simulink model "MultiLoop_mode3"  (Simulink 10.0)
settings: Solver=ode45  StartTime=0.0  StopTime=72  FixedStep=Ts_base  MinStep=1e-6  RelTol=1e-6
values from neighbouring files (symbols this model uses):
  xInitial = xFinal    [prepNextSimIteration.m]
undefined symbols (not defined in the file or in its folder): idv_init, integrator_init, r1_0, r4_0, seed, Ts_base, Ts_save, xmv_0
undefined symbols (not defined in the file): Eadj_0, r5_0, r7_0, setpoint_change_duration, setpoint_init, SP17_0
libraries: simulink x12, TElib x10
settings Model: Creator=ricker  LastModifiedBy=christopher
settings DataIOCC: LoadInitialState=on  SaveFinalState=on  SaveFormat=Structure  SignalLoggingSaveFormat=ModelDataLogs  SaveOutput=off  SaveTime=off  SignalLoggingName=sigsOut
settings OptimizationCC: InitFltsAndDblsToZero=on
settings DebuggingCC: SaveWithParameterizedLinksMsg=none  SignalResolutionControl=TryResolveAllWithWarning  MultiTaskDSMMsg=warning  MultiTaskCondExecSysMsg=none  FcnCallInpInsideContextMsg=warning
settings HardwareCC: TargetUnknown=on
settings GRTTargetCC: TargetFcnLib=ansi_tfl_tmw.mat  GeneratePreprocessorConditionals=Disable all
settings ConfigComp: CovExternalEMLEnable=off  CovSFcnEnable=off

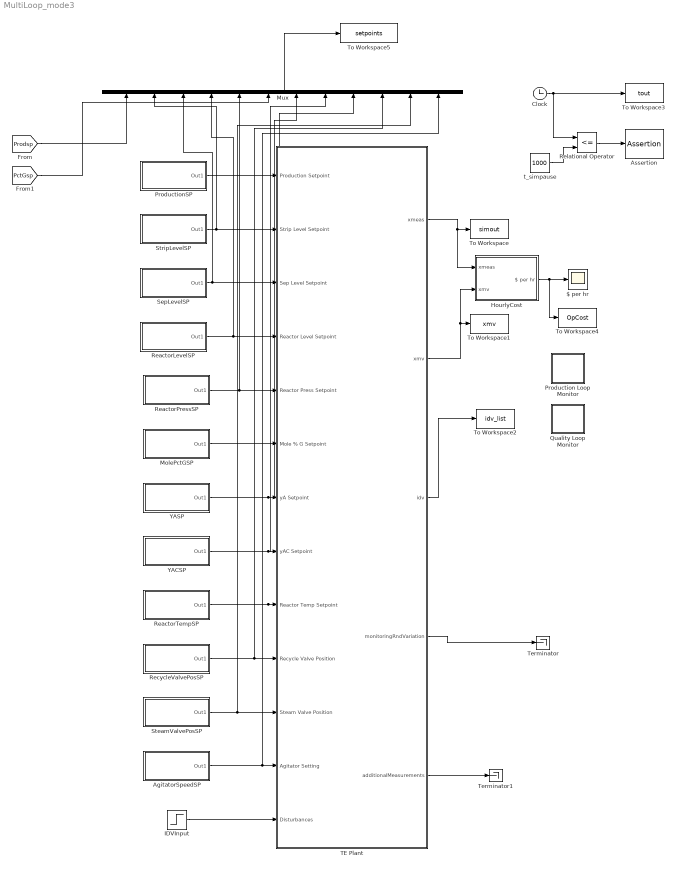
== system MultiLoop_mode3 ==
  $ per hr : Scope
  AgitatorSpeedSP : Subsystem  mask{SP_before=setpoint_init(1,12), SP_after=setpoint_init(2,12), tRampStart=setpoint_init(3,12), deltaT_ramp=setpoint_change_duration}
      mask prompts: SP_before "Value before ramp"; SP_after "Value after ramp"; tRampStart "Ramp start time"; deltaT_ramp "Ramp transition time"
  Assertion : Assertion  AssertionFailFcn=set_param(gcs ,'SimulationCommand','pause')  StopWhenAssertionFail=off
  Clock : Clock
  HourlyCost : Subsystem
  IDVInput : Step  Time=idv_init(3,:)  Before=idv_init(1,:)  After=idv_init(2,:)  SampleTime=0
  MolePctGSP : Subsystem  mask{SP_before=setpoint_init(1,6), SP_after=setpoint_init(2,6), tRampStart=setpoint_init(3,6), deltaT_ramp=setpoint_change_duration}
      mask prompts: SP_before "Value before ramp"; SP_after "Value after ramp"; tRampStart "Ramp start time"; deltaT_ramp "Ramp transition time"
  Mux : Mux  Inputs=12
  Production Loop Monitor : Subsystem
  ProductionSP : Subsystem  mask{SP_before=setpoint_init(1,1), SP_after=setpoint_init(2,1), tRampStart=setpoint_init(3,1), deltaT_ramp=setpoint_change_duration}
      mask prompts: SP_before "Value before ramp"; SP_after "Value after ramp"; tRampStart "Ramp start time"; deltaT_ramp "Ramp transition time"
  Quality Loop Monitor : Subsystem
  ReactorLevelSP : Subsystem  mask{SP_before=setpoint_init(1,4), SP_after=setpoint_init(2,4), tRampStart=setpoint_init(3,4), deltaT_ramp=setpoint_change_duration}
      mask prompts: SP_before "Value before ramp"; SP_after "Value after ramp"; tRampStart "Ramp start time"; deltaT_ramp "Ramp transition time"
  ReactorPressSP : Subsystem  mask{SP_before=setpoint_init(1,5), SP_after=setpoint_init(2,5), tRampStart=setpoint_init(3,5), deltaT_ramp=setpoint_change_duration}
      mask prompts: SP_before "Value before ramp"; SP_after "Value after ramp"; tRampStart "Ramp start time"; deltaT_ramp "Ramp transition time"
  ReactorTempSP : Subsystem  mask{SP_before=setpoint_init(1,9), SP_after=setpoint_init(2,9), tRampStart=setpoint_init(3,9), deltaT_ramp=setpoint_change_duration}
      mask prompts: SP_before "Value before ramp"; SP_after "Value after ramp"; tRampStart "Ramp start time"; deltaT_ramp "Ramp transition time"
  RecycleValvePosSP : Subsystem  mask{SP_before=setpoint_init(1,10), SP_after=setpoint_init(2,10), tRampStart=setpoint_init(3,10), deltaT_ramp=setpoint_change_duration}
      mask prompts: SP_before "Value before ramp"; SP_after "Value after ramp"; tRampStart "Ramp start time"; deltaT_ramp "Ramp transition time"
  Relational Operator : RelationalOperator  Operator=<=  OutDataTypeStr=boolean  RndMeth=Simplest
  SepLevelSP : Subsystem  mask{SP_before=setpoint_init(1,3), SP_after=setpoint_init(2,3), tRampStart=setpoint_init(3,3), deltaT_ramp=setpoint_change_duration}
      mask prompts: SP_before "Value before ramp"; SP_after "Value after ramp"; tRampStart "Ramp start time"; deltaT_ramp "Ramp transition time"
  SteamValvePosSP : Subsystem  mask{SP_before=setpoint_init(1,11), SP_after=setpoint_init(2,11), tRampStart=setpoint_init(3,11), deltaT_ramp=setpoint_change_duration}
      mask prompts: SP_before "Value before ramp"; SP_after "Value after ramp"; tRampStart "Ramp start time"; deltaT_ramp "Ramp transition time"
  StripLevelSP : Subsystem  mask{SP_before=setpoint_init(1,2), SP_after=setpoint_init(2,2), tRampStart=setpoint_init(3,2), deltaT_ramp=setpoint_change_duration}
      mask prompts: SP_before "Value before ramp"; SP_after "Value after ramp"; tRampStart "Ramp start time"; deltaT_ramp "Ramp transition time"
  TE Plant : Subsystem
  Terminator : Terminator
  Terminator1 : Terminator
  To Workspace : ToWorkspace  VariableName=simout  SampleTime=Ts_save
  To Workspace1 : ToWorkspace  VariableName=xmv  SampleTime=Ts_save
  To Workspace2 : ToWorkspace  VariableName=idv_list  SampleTime=Ts_save
  To Workspace3 : ToWorkspace  VariableName=tout  SampleTime=Ts_save
  To Workspace4 : ToWorkspace  VariableName=OpCost  SampleTime=Ts_save
  To Workspace5 : ToWorkspace  VariableName=setpoints  SampleTime=Ts_save
  YACSP : Subsystem  mask{SP_before=setpoint_init(1,8), SP_after=setpoint_init(2,8), tRampStart=setpoint_init(3,8), deltaT_ramp=setpoint_change_duration}
      mask prompts: SP_before "Value before ramp"; SP_after "Value after ramp"; tRampStart "Ramp start time"; deltaT_ramp "Ramp transition time"
  YASP : Subsystem  mask{SP_before=setpoint_init(1,7), SP_after=setpoint_init(2,7), tRampStart=setpoint_init(3,7), deltaT_ramp=setpoint_change_duration}
      mask prompts: SP_before "Value before ramp"; SP_after "Value after ramp"; tRampStart "Ramp start time"; deltaT_ramp "Ramp transition time"
  t_simpause : Constant  Value=1000
  wires:
  TE Plant/1(xmeas) -> HourlyCost/1(xmeas), To Workspace/1
  TE Plant/2(xmv) -> To Workspace1/1, HourlyCost/2(xmv)
  TE Plant/3(idv) -> To Workspace2/1
  Clock/1 -> Relational Operator/1, To Workspace3/1
  HourlyCost/1($ per hr) -> $ per hr/1, To Workspace4/1
  ProductionSP/1(Out1) -> TE Plant/1(Production Setpoint)
  AgitatorSpeedSP/1(Out1) -> Mux/12, TE Plant/12(Agitator Setting)
  SteamValvePosSP/1(Out1) -> Mux/11, TE Plant/11(Steam Valve Position)
  RecycleValvePosSP/1(Out1) -> Mux/10, TE Plant/10(Recycle Valve Position)
  ReactorTempSP/1(Out1) -> Mux/9, TE Plant/9(Reactor Temp Setpoint)
  YACSP/1(Out1) -> Mux/8, TE Plant/8(yAC Setpoint)
  YASP/1(Out1) -> Mux/7, TE Plant/7(yA Setpoint)
  MolePctGSP/1(Out1) -> TE Plant/6(Mole % G Setpoint)
  ReactorPressSP/1(Out1) -> TE Plant/5(Reactor Press Setpoint), Mux/5
  ReactorLevelSP/1(Out1) -> TE Plant/4(Reactor Level Setpoint), Mux/4
  SepLevelSP/1(Out1) -> TE Plant/3(Sep Level Setpoint), Mux/3
  StripLevelSP/1(Out1) -> TE Plant/2(Strip Level Setpoint), Mux/2
  IDVInput/1 -> TE Plant/13(Disturbances)
  Mux/1 -> To Workspace5/1
  TE Plant/4(monitoringRndVariation) -> Terminator/1
  TE Plant/5(additionalMeasurements) -> Terminator1/1
  [Prodsp] -> Mux/1
  [PctGsp] -> Mux/6
  Relational Operator/1 -> Assertion/1
  t_simpause/1 -> Relational Operator/2

== system MultiLoop_mode3/AgitatorSpeedSP ==
  Constant : Constant  Value=SP_before
  Constant1 : Constant  Value=deltaT_ramp
  Ramp : simulink/Sources/Ramp  slope=(SP_after-SP_before) /max(deltaT_ramp,0.1)  start=tRampStart  InitialOutput=0
  Saturation : Saturate  UpperLimit=max(SP_before, SP_after)  LowerLimit=min(SP_before, SP_after)
  Step : Step  Time=tRampStart  Before=SP_before  After=SP_after  SampleTime=0
  Sum : Sum  Inputs=|++
  Switch : Switch  Criteria=u2 > Threshold
  Out1 : Outport  VectorParamsAs1DForOutWhenUnconnected=off
  wires:
  Constant/1 -> Sum/1
  Ramp/1 -> Sum/2
  Sum/1 -> Saturation/1
  Constant1/1 -> Switch/2
  Switch/1 -> Out1/1
  Step/1 -> Switch/3
  Saturation/1 -> Switch/1

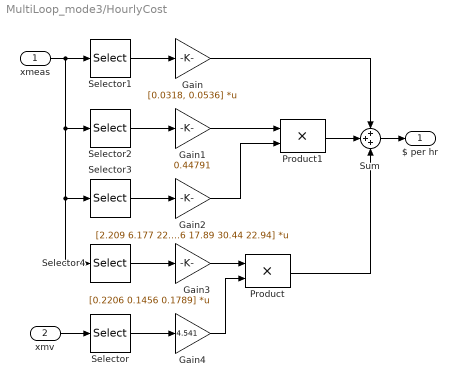
== system MultiLoop_mode3/HourlyCost ==
  xmeas : Inport  PortDimensions=41
  xmv : Inport  Port=2  PortDimensions=12
  Gain : Gain  Gain=[0.0318, 0.0536]  Multiplication=Matrix(K*u)  SaturateOnIntegerOverflow=on  OutDataTypeStr=Inherit: Same as input  ParamDataTypeStr=Inherit: Same as input
  Gain1 : Gain  Gain=0.44791  SaturateOnIntegerOverflow=on  OutDataTypeStr=Inherit: Same as input  ParamDataTypeStr=Inherit: Same as input
  Gain2 : Gain  Gain=[2.209 6.177 22.06 14.56 17.89 30.44 22.94]  Multiplication=Matrix(K*u)  SaturateOnIntegerOverflow=on  OutDataTypeStr=Inherit: Same as input  ParamDataTypeStr=Inherit: Same as input
  Gain3 : Gain  Gain=[0.2206 0.1456 0.1789]  Multiplication=Matrix(K*u)  SaturateOnIntegerOverflow=on  OutDataTypeStr=Inherit: Same as input  ParamDataTypeStr=Inherit: Same as input
  Gain4 : Gain  Gain=4.541  SaturateOnIntegerOverflow=on  OutDataTypeStr=Inherit: Same as input  ParamDataTypeStr=Inherit: Same as input
  Product : Product  SaturateOnIntegerOverflow=on  OutDataTypeStr=Inherit: Same as first input
  Product1 : Product  SaturateOnIntegerOverflow=on  OutDataTypeStr=Inherit: Same as first input
  Selector : Selector  InputPortWidth=12  IndexOptions=Index vector (dialog)  Indices=8  OutputSizes=1
  Selector1 : Selector  InputPortWidth=41  IndexOptions=Index vector (dialog)  Indices=[19 20]  OutputSizes=1
  Selector2 : Selector  InputPortWidth=41  IndexOptions=Index vector (dialog)  Indices=[10]  OutputSizes=1
  Selector3 : Selector  InputPortWidth=41  IndexOptions=Index vector (dialog)  Indices=[29, 31:36]  OutputSizes=1
  Selector4 : Selector  InputPortWidth=41  IndexOptions=Index vector (dialog)  Indices=[37:39]  OutputSizes=1
  Sum : Sum  Inputs=+++  SaturateOnIntegerOverflow=on
  $ per hr : Outport  VectorParamsAs1DForOutWhenUnconnected=off
  wires:
  xmv/1 -> Selector/1
  xmeas/1 -> Selector1/1, Selector2/1, Selector3/1, Selector4/1
  Selector1/1 -> Gain/1
  Selector2/1 -> Gain1/1
  Selector3/1 -> Gain2/1
  Selector4/1 -> Gain3/1
  Selector/1 -> Gain4/1
  Gain3/1 -> Product/1
  Gain4/1 -> Product/2
  Sum/1 -> $ per hr/1
  Product/1 -> Sum/3
  Gain/1 -> Sum/1
  Product1/1 -> Sum/2
  Gain1/1 -> Product1/1
  Gain2/1 -> Product1/2

== system MultiLoop_mode3/MolePctGSP ==
  Constant : Constant  Value=SP_before
  Constant1 : Constant  Value=deltaT_ramp
  Ramp : simulink/Sources/Ramp  slope=(SP_after-SP_before) /max(deltaT_ramp,0.1)  start=tRampStart  InitialOutput=0
  Saturation1 : Saturate  UpperLimit=max(SP_before, SP_after)  LowerLimit=min(SP_before, SP_after)
  Step : Step  Time=tRampStart  Before=SP_before  After=SP_after  SampleTime=0
  Sum : Sum  Inputs=|++
  Switch : Switch  Criteria=u2 > Threshold
  Out1 : Outport  VectorParamsAs1DForOutWhenUnconnected=off
  wires:
  Constant/1 -> Sum/1
  Ramp/1 -> Sum/2
  Sum/1 -> Saturation1/1
  Constant1/1 -> Switch/2
  Switch/1 -> Out1/1
  Step/1 -> Switch/3
  Saturation1/1 -> Switch/1

== system MultiLoop_mode3/Production Loop Monitor ==
  Mux2 : Mux  Inputs=2
  Production : Scope
  wires:
  Mux2/1 -> Production/1
  [xmeas17] -> Mux2/2
  [Prodsp] -> Mux2/1

== system MultiLoop_mode3/ProductionSP ==
  Constant : Constant  Value=SP_before
  Constant1 : Constant  Value=deltaT_ramp
  Ramp : simulink/Sources/Ramp  slope=(SP_after-SP_before) /max(deltaT_ramp,0.1)  start=tRampStart  InitialOutput=0
  Saturation : Saturate  UpperLimit=max(SP_before, SP_after)  LowerLimit=min(SP_before, SP_after)
  Step : Step  Time=tRampStart  Before=SP_before  After=SP_after  SampleTime=0
  Sum : Sum  Inputs=|++
  Switch : Switch  Criteria=u2 > Threshold
  Out1 : Outport  VectorParamsAs1DForOutWhenUnconnected=off
  wires:
  Constant/1 -> Sum/1
  Ramp/1 -> Sum/2
  Sum/1 -> Saturation/1
  Constant1/1 -> Switch/2
  Switch/1 -> Out1/1
  Step/1 -> Switch/3
  Saturation/1 -> Switch/1

== system MultiLoop_mode3/Quality Loop Monitor ==
  Mux2 : Mux  Inputs=2
  Quality : Scope
  wires:
  [PctGsp] -> Mux2/1
  [xmeas40] -> Mux2/2
  Mux2/1 -> Quality/1

== system MultiLoop_mode3/ReactorLevelSP ==
  Constant : Constant  Value=SP_before
  Constant1 : Constant  Value=deltaT_ramp
  Ramp : simulink/Sources/Ramp  slope=(SP_after-SP_before) /max(deltaT_ramp,0.1)  start=tRampStart  InitialOutput=0
  Saturation : Saturate  UpperLimit=max(SP_before, SP_after)  LowerLimit=min(SP_before, SP_after)
  Step : Step  Time=tRampStart  Before=SP_before  After=SP_after  SampleTime=0
  Sum : Sum  Inputs=|++
  Switch : Switch  Criteria=u2 > Threshold
  Out1 : Outport  VectorParamsAs1DForOutWhenUnconnected=off
  wires:
  Constant/1 -> Sum/1
  Ramp/1 -> Sum/2
  Sum/1 -> Saturation/1
  Constant1/1 -> Switch/2
  Switch/1 -> Out1/1
  Step/1 -> Switch/3
  Saturation/1 -> Switch/1

== system MultiLoop_mode3/ReactorPressSP ==
  Constant : Constant  Value=SP_before
  Constant1 : Constant  Value=deltaT_ramp
  Ramp : simulink/Sources/Ramp  slope=(SP_after-SP_before) /max(deltaT_ramp,0.1)  start=tRampStart  InitialOutput=0
  Saturation1 : Saturate  UpperLimit=max(SP_before, SP_after)  LowerLimit=min(SP_before, SP_after)
  Step : Step  Time=tRampStart  Before=SP_before  After=SP_after  SampleTime=0
  Sum : Sum  Inputs=|++
  Switch : Switch  Criteria=u2 > Threshold
  Out1 : Outport  VectorParamsAs1DForOutWhenUnconnected=off
  wires:
  Constant/1 -> Sum/1
  Ramp/1 -> Sum/2
  Sum/1 -> Saturation1/1
  Constant1/1 -> Switch/2
  Switch/1 -> Out1/1
  Step/1 -> Switch/3
  Saturation1/1 -> Switch/1

== system MultiLoop_mode3/ReactorTempSP ==
  Constant : Constant  Value=SP_before
  Constant1 : Constant  Value=deltaT_ramp
  Ramp : simulink/Sources/Ramp  slope=(SP_after-SP_before) /max(deltaT_ramp,0.1)  start=tRampStart  InitialOutput=0
  Saturation1 : Saturate  UpperLimit=max(SP_before, SP_after)  LowerLimit=min(SP_before, SP_after)
  Step : Step  Time=tRampStart  Before=SP_before  After=SP_after  SampleTime=0
  Sum : Sum  Inputs=|++
  Switch : Switch  Criteria=u2 > Threshold
  Out1 : Outport  VectorParamsAs1DForOutWhenUnconnected=off
  wires:
  Constant/1 -> Sum/1
  Ramp/1 -> Sum/2
  Sum/1 -> Saturation1/1
  Constant1/1 -> Switch/2
  Switch/1 -> Out1/1
  Step/1 -> Switch/3
  Saturation1/1 -> Switch/1

== system MultiLoop_mode3/RecycleValvePosSP ==
  Constant : Constant  Value=SP_before
  Constant1 : Constant  Value=deltaT_ramp
  Ramp : simulink/Sources/Ramp  slope=(SP_after-SP_before) /max(deltaT_ramp,0.1)  start=tRampStart  InitialOutput=0
  Saturation1 : Saturate  UpperLimit=max(SP_before, SP_after)  LowerLimit=min(SP_before, SP_after)
  Step : Step  Time=tRampStart  Before=SP_before  After=SP_after  SampleTime=0
  Sum : Sum  Inputs=|++
  Switch : Switch  Criteria=u2 > Threshold
  Out1 : Outport  VectorParamsAs1DForOutWhenUnconnected=off
  wires:
  Constant/1 -> Sum/1
  Ramp/1 -> Sum/2
  Sum/1 -> Saturation1/1
  Constant1/1 -> Switch/2
  Switch/1 -> Out1/1
  Step/1 -> Switch/3
  Saturation1/1 -> Switch/1

== system MultiLoop_mode3/SepLevelSP ==
  Constant : Constant  Value=SP_before
  Constant1 : Constant  Value=deltaT_ramp
  Ramp : simulink/Sources/Ramp  slope=(SP_after-SP_before) /max(deltaT_ramp,0.1)  start=tRampStart  InitialOutput=0
  Saturation1 : Saturate  UpperLimit=max(SP_before, SP_after)  LowerLimit=min(SP_before, SP_after)
  Step : Step  Time=tRampStart  Before=SP_before  After=SP_after  SampleTime=0
  Sum : Sum  Inputs=|++
  Switch : Switch  Criteria=u2 > Threshold
  Out1 : Outport  VectorParamsAs1DForOutWhenUnconnected=off
  wires:
  Constant/1 -> Sum/1
  Ramp/1 -> Sum/2
  Sum/1 -> Saturation1/1
  Constant1/1 -> Switch/2
  Switch/1 -> Out1/1
  Step/1 -> Switch/3
  Saturation1/1 -> Switch/1

== system MultiLoop_mode3/SteamValvePosSP ==
  Constant : Constant  Value=SP_before
  Constant1 : Constant  Value=deltaT_ramp
  Ramp : simulink/Sources/Ramp  slope=(SP_after-SP_before) /max(deltaT_ramp,0.1)  start=tRampStart  InitialOutput=0
  Saturation1 : Saturate  UpperLimit=max(SP_before, SP_after)  LowerLimit=min(SP_before, SP_after)
  Step : Step  Time=tRampStart  Before=SP_before  After=SP_after  SampleTime=0
  Sum : Sum  Inputs=|++
  Switch : Switch  Criteria=u2 > Threshold
  Out1 : Outport  VectorParamsAs1DForOutWhenUnconnected=off
  wires:
  Constant/1 -> Sum/1
  Ramp/1 -> Sum/2
  Sum/1 -> Saturation1/1
  Constant1/1 -> Switch/2
  Switch/1 -> Out1/1
  Step/1 -> Switch/3
  Saturation1/1 -> Switch/1

== system MultiLoop_mode3/StripLevelSP ==
  Constant : Constant  Value=SP_before
  Constant1 : Constant  Value=deltaT_ramp
  Ramp : simulink/Sources/Ramp  slope=(SP_after-SP_before) /max(deltaT_ramp,0.1)  start=tRampStart  InitialOutput=0
  Saturation : Saturate  UpperLimit=max(SP_before, SP_after)  LowerLimit=min(SP_before, SP_after)
  Step : Step  Time=tRampStart  Before=SP_before  After=SP_after  SampleTime=0
  Sum : Sum  Inputs=|++
  Switch : Switch  Criteria=u2 > Threshold
  Out1 : Outport  VectorParamsAs1DForOutWhenUnconnected=off
  wires:
  Constant/1 -> Sum/1
  Ramp/1 -> Sum/2
  Sum/1 -> Saturation/1
  Constant1/1 -> Switch/2
  Switch/1 -> Out1/1
  Step/1 -> Switch/3
  Saturation/1 -> Switch/1

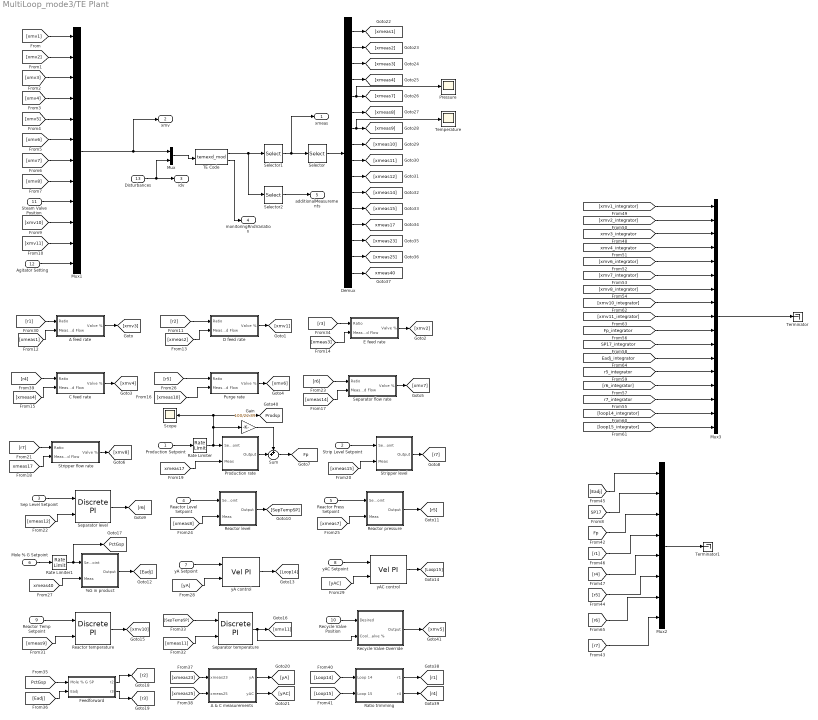
== system MultiLoop_mode3/TE Plant ==
  Production Setpoint : Inport
  Strip Level Setpoint : Inport  Port=2
  Sep Level Setpoint : Inport  Port=3
  Reactor Level Setpoint : Inport  Port=4
  Reactor Press Setpoint : Inport  Port=5
  Mole % G Setpoint : Inport  Port=6
  yA Setpoint : Inport  Port=7
  yAC Setpoint : Inport  Port=8
  Reactor Temp Setpoint : Inport  Port=9
  Recycle Valve Position : Inport  Port=10
  Steam Valve Position : Inport  Port=11
  Agitator Setting : Inport  Port=12
  Disturbances : Inport  Port=13
  %G in product : Subsystem  AncestorBlock=TElib/Discrete PI  mask{Kc=-0.4, Ti=100/60, Ts=Ts_base, x0=Eadj_0, Hi=inf, Lo=-inf}
  A & C measurements : Subsystem
  A feed rate : Subsystem
  C feed rate : Subsystem
  D feed rate : Subsystem
  Demux : Demux  Outputs=16
  E feed rate : Subsystem
  Feedforward : Subsystem
  Gain : Gain  Gain=100/22.89  SaturateOnIntegerOverflow=on  OutDataTypeStr=Inherit: Same as input  ParamDataTypeStr=Inherit: Same as input
  Mux : Mux  Inputs=2
  Mux1 : Mux  Inputs=12
  Mux2 : Mux  Inputs=8
  Mux3 : Mux  Inputs=17
  Pressure : Scope
  Production rate : Subsystem  AncestorBlock=TElib/Discrete PI  mask{Kc=3.2, Ti=120/60, Ts=Ts_base, x0=0, Hi=30, Lo=-30}
  Purge rate : Subsystem
  Rate Limiter : RateLimiter  RisingSlewLimit=0.3*22.95/24  FallingSlewLimit=-0.3*22.95/24
  Rate Limiter1 : RateLimiter  RisingSlewLimit=50/24  FallingSlewLimit=-50/24
  Ratio trimming : Subsystem
  Reactor level : Subsystem  AncestorBlock=TElib/Discrete PI  mask{Kc=0.8, Ti=60/60, Ts=Ts_base, x0=SP17_0, Hi=120, Lo=0}
  Reactor pressure : Subsystem  AncestorBlock=TElib/Discrete PI  mask{Kc=-1e-4, Ti=20/60, Ts=Ts_base, x0=r5_0, Hi=100, Lo=0}
  Reactor temperature : TElib/Discrete PI  Kc=-8  Ti=7.5/60  Ts=Ts_base  x0=xmv_0(10)  Hi=100  Lo=0
      link override Vel PI/Goto: GotoTag=xmv10_integrator
      link override Vel PI/Unit Delay: InitialCondition=integrator_init(8)
  Recycle Valve Override : Subsystem  AncestorBlock=TElib/Discrete PI
  Scope : Scope
  Selector : Selector  InputPortWidth=41  IndexOptions=Index vector (dialog)  Indices=[1:4, 7:12, 14, 15, 17, 23, 25, 40]  OutputSizes=1
  Selector1 : Selector  InputPortWidth=73  IndexOptions=Index vector (dialog)  Indices=[1:41]  OutputSizes=1
  Selector2 : Selector  InputPortWidth=73  IndexOptions=Index vector (dialog)  Indices=[42:73]  OutputSizes=1
  Separator flow rate : Subsystem
  Separator level : TElib/Discrete PI  Kc=-1e-3  Ti=200/60  Ts=Ts_base  x0=r6_0  Hi=100  Lo=0
      link override Vel PI/Goto: GotoTag=r6_integrator
      link override Vel PI/Unit Delay: InitialCondition=integrator_init(14)
  Separator temperature : TElib/Discrete PI  Kc=-4  Ti=15/60  Ts=Ts_base  x0=xmv_0(11)  Hi=100  Lo=0
      link override Vel PI/Goto: GotoTag=xmv11_integrator
      link override Vel PI/Unit Delay: InitialCondition=integrator_init(9)
  Stripper flow rate : Subsystem
  Stripper level : Subsystem  AncestorBlock=TElib/Discrete PI  mask{Kc=-2e-4, Ti=200/60, Ts=Ts_base, x0=r7_0, Hi=100, Lo=0}
  Sum : Sum  Inputs=++|  SaturateOnIntegerOverflow=on
  TE Code : S-Function  FunctionName=temexd_mod  Parameters=xInitial.signals(1).values,seed,243  SFunctionDeploymentMode=off  EnableBusSupport=off
  Temperature : Scope
  Terminator : Terminator
  Terminator1 : Terminator
  yA control : TElib/Discrete PI/Vel PI  Kc=2e-4  Ti=1  Ts=0.1
      link override Goto: GotoTag=loop14_integrator
      link override Unit Delay: InitialCondition=integrator_init(16)
  yAC control : TElib/Discrete PI/Vel PI  Kc=3e-4  Ti=2  Ts=0.1
      link override Goto: GotoTag=loop15_integrator
      link override Unit Delay: InitialCondition=integrator_init(17)
  xmeas : Outport  VectorParamsAs1DForOutWhenUnconnected=off
  xmv : Outport  Port=2  VectorParamsAs1DForOutWhenUnconnected=off
  idv : Outport  Port=3  VectorParamsAs1DForOutWhenUnconnected=off
  monitoringRndVariation : Outport  Port=4  VectorParamsAs1DForOutWhenUnconnected=off
  additionalMeasurements : Outport  Port=5  VectorParamsAs1DForOutWhenUnconnected=off
  tag scope: Fp=global, PctGsp=global, Prodsp=global, xmeas17=global, xmeas40=global
  wires:
  Mux/1 -> TE Code/1
  Disturbances/1 -> Mux/2, idv/1
  TE Code/1 -> Selector2/1, Selector1/1
  [xmv1] -> Mux1/1
  [xmv2] -> Mux1/2
  [xmv3] -> Mux1/3
  [xmv4] -> Mux1/4
  [xmv6] -> Mux1/6
  [xmv7] -> Mux1/7
  [xmv8] -> Mux1/8
  Steam Valve Position/1 -> Mux1/9
  [xmv10] -> Mux1/10
  [xmv11] -> Mux1/11
  Agitator Setting/1 -> Mux1/12
  A feed rate/1(Valve %) -> [xmv3]
  [xmeas1] -> A feed rate/2(Measured Flow)
  D feed rate/1(Valve %) -> [xmv1]
  [xmeas2] -> D feed rate/2(Measured Flow)
  E feed rate/1(Valve %) -> [xmv2]
  [xmeas3] -> E feed rate/2(Measured Flow)
  C feed rate/1(Valve %) -> [xmv4]
  [xmeas4] -> C feed rate/2(Measured Flow)
  Purge rate/1(Valve %) -> [xmv6]
  [xmeas10] -> Purge rate/2(Measured Flow)
  Separator flow rate/1(Valve %) -> [xmv7]
  [xmeas14] -> Separator flow rate/2(Measured Flow)
  Stripper flow rate/1(Valve %) -> [xmv8]
  [xmeas17] -> Stripper flow rate/2(Measured Flow)
  [xmeas17] -> Production rate/2(Meas)
  [xmeas15] -> Stripper level/2(Meas)
  Strip Level Setpoint/1 -> Stripper level/1(Setpoint)
  Stripper level/1(Output) -> [r7]
  [r7] -> Stripper flow rate/1(Ratio)
  [xmeas12] -> Separator level/2
  Sep Level Setpoint/1 -> Separator level/1
  Separator level/1 -> [r6]
  [r6] -> Separator flow rate/1(Ratio)
  [xmeas8] -> Reactor level/2(Meas)
  Reactor Level Setpoint/1 -> Reactor level/1(Setpoint)
  Reactor level/1(Output) -> [SepTempSP]
  [xmeas7] -> Reactor pressure/2(Meas)
  Reactor Press Setpoint/1 -> Reactor pressure/1(Setpoint)
  Reactor pressure/1(Output) -> [r5]
  [r5] -> Purge rate/1(Ratio)
  [xmeas40] -> %G in product/2(Meas)
  %G in product/1(Output) -> [Eadj]
  [yA] -> yA control/2
  yA Setpoint/1 -> yA control/1
  yA control/1 -> [Loop14]
  [yAC] -> yAC control/2
  yAC Setpoint/1 -> yAC control/1
  yAC control/1 -> [Loop15]
  [r1] -> A feed rate/1(Ratio)
  [xmeas9] -> Reactor temperature/2
  Reactor Temp Setpoint/1 -> Reactor temperature/1
  Reactor temperature/1 -> [xmv10]
  [xmeas11] -> Separator temperature/2
  [SepTempSP] -> Separator temperature/1
  Separator temperature/1 -> [xmv11], Recycle Valve Override/2(Coolant Valve %)
  [r2] -> D feed rate/1(Ratio)
  [r3] -> E feed rate/1(Ratio)
  [PctGsp] -> Feedforward/1(Mole % G SP)
  [Eadj] -> Feedforward/2(Eadj)
  Feedforward/1(r2) -> [r2]
  Feedforward/2(r3) -> [r3]
  [xmeas23] -> A & C measurements/1(xmeas23)
  [xmeas25] -> A & C measurements/2(xmeas25)
  A & C measurements/1(yA) -> [yA]
  A & C measurements/2(yAC) -> [yAC]
  Mux1/1 -> Mux/1, xmv/1
  Selector/1 -> Demux/1
  Demux/1 -> [xmeas1]
  Demux/2 -> [xmeas2]
  Demux/3 -> [xmeas3]
  Demux/4 -> [xmeas4]
  Demux/5 -> [xmeas7], Pressure/1
  Demux/6 -> [xmeas8]
  Demux/7 -> [xmeas9], Temperature/1
  Demux/8 -> [xmeas10]
  Demux/9 -> [xmeas11]
  Demux/10 -> [xmeas12]
  Demux/11 -> [xmeas14]
  Demux/12 -> [xmeas15]
  Demux/13 -> [xmeas17]
  Demux/14 -> [xmeas23]
  Demux/15 -> [xmeas25]
  Demux/16 -> [xmeas40]
  [r4] -> C feed rate/1(Ratio)
  [Loop14] -> Ratio trimming/1(Loop 14)
  [Loop15] -> Ratio trimming/2(Loop 15)
  Ratio trimming/1(r1) -> [r1]
  Ratio trimming/2(r4) -> [r4]
  Production Setpoint/1 -> Rate Limiter/1
  Rate Limiter/1 -> Production rate/1(Setpoint), Scope/1, [Prodsp], Gain/1
  Mole % G Setpoint/1 -> Rate Limiter1/1
  Rate Limiter1/1 -> %G in product/1(Setpoint), [PctGsp]
  Production rate/1(Output) -> Sum/2
  Sum/1 -> [Fp]
  Gain/1 -> Sum/1
  [xmv5] -> Mux1/5
  Recycle Valve Override/1(Output) -> [xmv5]
  Recycle Valve Position/1 -> Recycle Valve Override/1(Desired)
  Selector2/1 -> additionalMeasurements/1
  TE Code/2 -> monitoringRndVariation/1
  Selector1/1 -> xmeas/1, Selector/1
  [Eadj] -> Mux2/1
  [SP17] -> Mux2/2
  [Fp] -> Mux2/3
  [r1] -> Mux2/4
  [r4] -> Mux2/5
  [r5] -> Mux2/6
  [r7] -> Mux2/8
  [xmv1_integrator] -> Mux3/1
  [xmv2_integrator] -> Mux3/2
  [xmv3_integrator] -> Mux3/3
  [xmv4_integrator] -> Mux3/4
  [xmv6_integrator] -> Mux3/5
  [xmv7_integrator] -> Mux3/6
  [xmv8_integrator] -> Mux3/7
  [xmv10_integrator] -> Mux3/8
  [xmv11_integrator] -> Mux3/9
  [Fp_integrator] -> Mux3/10
  [SP17_integrator] -> Mux3/11
  [Eadj_integrator] -> Mux3/12
  [r5_integrator] -> Mux3/13
  [r6_integrator] -> Mux3/14
  [r7_integrator] -> Mux3/15
  [loop14_integrator] -> Mux3/16
  [loop15_integrator] -> Mux3/17
  [r6] -> Mux2/7
  Mux3/1 -> Terminator/1
  Mux2/1 -> Terminator1/1

== system MultiLoop_mode3/YACSP ==
  Constant : Constant  Value=SP_before
  Constant1 : Constant  Value=deltaT_ramp
  Ramp : simulink/Sources/Ramp  slope=(SP_after-SP_before) /max(deltaT_ramp,0.1)  start=tRampStart  InitialOutput=0
  Saturation1 : Saturate  UpperLimit=max(SP_before, SP_after)  LowerLimit=min(SP_before, SP_after)
  Step : Step  Time=tRampStart  Before=SP_before  After=SP_after  SampleTime=0
  Sum : Sum  Inputs=|++
  Switch : Switch  Criteria=u2 > Threshold
  Out1 : Outport  VectorParamsAs1DForOutWhenUnconnected=off
  wires:
  Constant/1 -> Sum/1
  Ramp/1 -> Sum/2
  Sum/1 -> Saturation1/1
  Constant1/1 -> Switch/2
  Switch/1 -> Out1/1
  Step/1 -> Switch/3
  Saturation1/1 -> Switch/1

== system MultiLoop_mode3/YASP ==
  Constant : Constant  Value=SP_before
  Constant1 : Constant  Value=deltaT_ramp
  Ramp : simulink/Sources/Ramp  slope=(SP_after-SP_before) /max(deltaT_ramp,0.1)  start=tRampStart  InitialOutput=0
  Saturation1 : Saturate  UpperLimit=max(SP_before, SP_after)  LowerLimit=min(SP_before, SP_after)
  Step : Step  Time=tRampStart  Before=SP_before  After=SP_after  SampleTime=0
  Sum : Sum  Inputs=|++
  Switch : Switch  Criteria=u2 > Threshold
  Out1 : Outport  VectorParamsAs1DForOutWhenUnconnected=off
  wires:
  Constant/1 -> Sum/1
  Ramp/1 -> Sum/2
  Sum/1 -> Saturation1/1
  Constant1/1 -> Switch/2
  Switch/1 -> Out1/1
  Step/1 -> Switch/3
  Saturation1/1 -> Switch/1

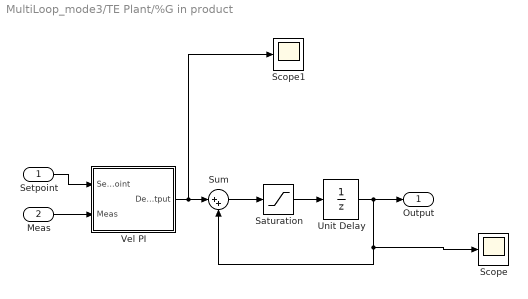
== system MultiLoop_mode3/TE Plant/%G in product ==
  Setpoint : Inport
  Meas : Inport  Port=2
  Saturation : Saturate  UpperLimit=Hi  LowerLimit=Lo
  Scope : Scope
  Scope1 : Scope
  Sum : Sum  Inputs=|++  SaturateOnIntegerOverflow=on
  Unit Delay : UnitDelay  InitialCondition=x0  SampleTime=Ts
  Vel PI : Subsystem  mask{Kc=Kc, Ti=Ti, Ts=Ts}
  Output : Outport
  wires:
  Setpoint/1 -> Vel PI/1(Setpoint)
  Meas/1 -> Vel PI/2(Meas)
  Unit Delay/1 -> Output/1, Scope/1, Sum/2
  Saturation/1 -> Unit Delay/1
  Vel PI/1(Delta Output) -> Scope1/1, Sum/1
  Sum/1 -> Saturation/1

== system MultiLoop_mode3/TE Plant/A & C measurements ==
  xmeas23 : Inport
  xmeas25 : Inport  Port=2
  Gain1 : Gain  Gain=100  SaturateOnIntegerOverflow=on  OutDataTypeStr=Inherit: Same as input  ParamDataTypeStr=Inherit: Same as input
  Product1 : Product  Inputs=*/  SaturateOnIntegerOverflow=on  OutDataTypeStr=Inherit: Same as first input
  Sum1 : Sum  Inputs=++|  SaturateOnIntegerOverflow=on
  yA : Outport  VectorParamsAs1DForOutWhenUnconnected=off
  yAC : Outport  Port=2  VectorParamsAs1DForOutWhenUnconnected=off
  wires:
  Sum1/1 -> yAC/1, Product1/2
  xmeas23/1 -> Sum1/1, Gain1/1
  xmeas25/1 -> Sum1/2
  Gain1/1 -> Product1/1
  Product1/1 -> yA/1

== system MultiLoop_mode3/TE Plant/A feed rate ==
  Ratio : Inport
  Measured Flow : Inport  Port=2
  Discrete PI : Subsystem  AncestorBlock=TElib/Discrete PI  mask{Kc=0.01, Ti=0.001/60, Ts=Ts_base, x0=xmv_0(3), Hi=100, Lo=0}
  Product : Product  SaturateOnIntegerOverflow=on  OutDataTypeStr=Inherit: Same as first input
  Scope : Scope
  Valve % : Outport  VectorParamsAs1DForOutWhenUnconnected=off
  wires:
  Discrete PI/1(Output) -> Valve %/1
  Ratio/1 -> Product/1
  [Fp] -> Product/2
  Measured Flow/1 -> Discrete PI/2(Meas)
  Product/1 -> Scope/1, Discrete PI/1(Setpoint)

== system MultiLoop_mode3/TE Plant/C feed rate ==
  Ratio : Inport
  Measured Flow : Inport  Port=2
  Discrete PI : Subsystem  AncestorBlock=TElib/Discrete PI  mask{Kc=0.003, Ti=0.001/60, Ts=Ts_base, x0=xmv_0(4), Hi=100, Lo=0}
  Product : Product  SaturateOnIntegerOverflow=on  OutDataTypeStr=Inherit: Same as first input
  Scope : Scope  NumInputPorts=2
  Valve % : Outport  VectorParamsAs1DForOutWhenUnconnected=off
  wires:
  Product/1 -> Scope/1, Discrete PI/1(Setpoint)
  Measured Flow/1 -> Scope/2, Discrete PI/2(Meas)
  [Fp] -> Product/2
  Ratio/1 -> Product/1
  Discrete PI/1(Output) -> Valve %/1

== system MultiLoop_mode3/TE Plant/D feed rate ==
  Ratio : Inport
  Measured Flow : Inport  Port=2
  Discrete PI : TElib/Discrete PI  Kc=1.6e-6  Ti=0.001/60  Ts=Ts_base  x0=xmv_0(1)  Hi=100  Lo=0
      link override Vel PI/Goto: GotoTag=xmv1_integrator
      link override Vel PI/Unit Delay: InitialCondition=integrator_init(1)
  Product : Product  SaturateOnIntegerOverflow=on  OutDataTypeStr=Inherit: Same as first input
  Valve % : Outport  VectorParamsAs1DForOutWhenUnconnected=off
  wires:
  Product/1 -> Discrete PI/1
  Measured Flow/1 -> Discrete PI/2
  [Fp] -> Product/2
  Ratio/1 -> Product/1
  Discrete PI/1 -> Valve %/1

== system MultiLoop_mode3/TE Plant/E feed rate ==
  Ratio : Inport
  Measured Flow : Inport  Port=2
  Discrete PI : TElib/Discrete PI  Kc=1.8e-6  Ti=0.001/60  Ts=Ts_base  x0=xmv_0(2)  Hi=100  Lo=0
      link override Vel PI/Goto: GotoTag=xmv2_integrator
      link override Vel PI/Unit Delay: InitialCondition=integrator_init(2)
  Product : Product  SaturateOnIntegerOverflow=on  OutDataTypeStr=Inherit: Same as first input
  Valve % : Outport  VectorParamsAs1DForOutWhenUnconnected=off
  wires:
  Product/1 -> Discrete PI/1
  Measured Flow/1 -> Discrete PI/2
  [Fp] -> Product/2
  Ratio/1 -> Product/1
  Discrete PI/1 -> Valve %/1

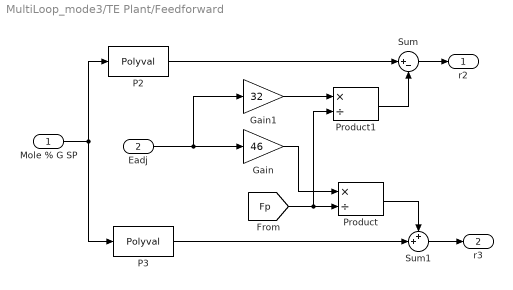
== system MultiLoop_mode3/TE Plant/Feedforward ==
  Mole % G SP : Inport
  Eadj : Inport  Port=2
  Gain : Gain  Gain=46  SaturateOnIntegerOverflow=on  OutDataTypeStr=Inherit: Same as input  ParamDataTypeStr=Inherit: Same as input
  Gain1 : Gain  Gain=32  SaturateOnIntegerOverflow=on  OutDataTypeStr=Inherit: Same as input  ParamDataTypeStr=Inherit: Same as input
  P2 : Polyval  Coefs="[1.5192e-003  5.9446e-001  2.7690e-001]"
  P3 : Polyval  Coefs="[-1.1377e-003 -8.0893e-001  9.1060e+001]"
  Product : Product  Inputs=*/  SaturateOnIntegerOverflow=on  OutDataTypeStr=Inherit: Same as first input
  Product1 : Product  Inputs=*/  SaturateOnIntegerOverflow=on  OutDataTypeStr=Inherit: Same as first input
  Sum : Sum  Inputs=|+-  SaturateOnIntegerOverflow=on
  Sum1 : Sum  Inputs=++|  SaturateOnIntegerOverflow=on
  r2 : Outport  VectorParamsAs1DForOutWhenUnconnected=off
  r3 : Outport  Port=2  VectorParamsAs1DForOutWhenUnconnected=off
  wires:
  Mole % G SP/1 -> P2/1, P3/1
  Sum/1 -> r2/1
  P2/1 -> Sum/1
  Sum1/1 -> r3/1
  P3/1 -> Sum1/2
  Product/1 -> Sum1/1
  [Fp] -> Product/2, Product1/2
  Gain/1 -> Product/1
  Eadj/1 -> Gain/1, Gain1/1
  Product1/1 -> Sum/2
  Gain1/1 -> Product1/1

== system MultiLoop_mode3/TE Plant/Production rate ==
  Setpoint : Inport
  Meas : Inport  Port=2
  Saturation : Saturate  UpperLimit=Hi  LowerLimit=Lo
  Sum : Sum  Inputs=|++  SaturateOnIntegerOverflow=on
  Unit Delay : UnitDelay  InitialCondition=x0  SampleTime=Ts
  Vel PI : Subsystem  mask{Kc=Kc, Ti=Ti, Ts=Ts}
  Output : Outport
  wires:
  Setpoint/1 -> Vel PI/1(Setpoint)
  Meas/1 -> Vel PI/2(Meas)
  Unit Delay/1 -> Output/1, Sum/2
  Saturation/1 -> Unit Delay/1
  Vel PI/1(Delta Output) -> Sum/1
  Sum/1 -> Saturation/1

== system MultiLoop_mode3/TE Plant/Purge rate ==
  Ratio : Inport
  Measured Flow : Inport  Port=2
  Discrete PI : TElib/Discrete PI  Kc=0.01  Ti=0.001/60  Ts=Ts_base  x0=xmv_0(6)  Hi=100  Lo=0
      link override Vel PI/Goto: GotoTag=xmv6_integrator
      link override Vel PI/Unit Delay: InitialCondition=integrator_init(5)
  Product : Product  SaturateOnIntegerOverflow=on  OutDataTypeStr=Inherit: Same as first input
  Valve % : Outport  VectorParamsAs1DForOutWhenUnconnected=off
  wires:
  Discrete PI/1 -> Valve %/1
  Ratio/1 -> Product/1
  [Fp] -> Product/2
  Measured Flow/1 -> Discrete PI/2
  Product/1 -> Discrete PI/1

== system MultiLoop_mode3/TE Plant/Ratio trimming ==
  Loop 14 : Inport
  Loop 15 : Inport  Port=2
  Sum1 : Sum  Inputs=-++  SaturateOnIntegerOverflow=on
  Sum2 : Sum  Inputs=++|  SaturateOnIntegerOverflow=on
  Unit Delay : UnitDelay  InitialCondition=r1_0  SampleTime=0.1  HasFrameUpgradeWarning=on
  Unit Delay1 : UnitDelay  InitialCondition=r4_0  SampleTime=0.1  HasFrameUpgradeWarning=on
  r1 : Outport  VectorParamsAs1DForOutWhenUnconnected=off
  r4 : Outport  Port=2  VectorParamsAs1DForOutWhenUnconnected=off
  wires:
  Loop 15/1 -> Sum1/2
  Unit Delay/1 -> Sum2/1
  Unit Delay1/1 -> Sum1/3
  Sum2/1 -> Unit Delay/1, r1/1
  Loop 14/1 -> Sum2/2, Sum1/1
  Sum1/1 -> Unit Delay1/1, r4/1

== system MultiLoop_mode3/TE Plant/Reactor level ==
  Setpoint : Inport
  Meas : Inport  Port=2
  Saturation : Saturate  UpperLimit=Hi  LowerLimit=Lo
  Sum : Sum  Inputs=|++  SaturateOnIntegerOverflow=on
  Unit Delay : UnitDelay  InitialCondition=x0  SampleTime=Ts
  Vel PI : Subsystem  mask{Kc=Kc, Ti=Ti, Ts=Ts}
  Output : Outport
  tag scope: SP17=global
  wires:
  Setpoint/1 -> Vel PI/1(Setpoint)
  Meas/1 -> Vel PI/2(Meas)
  Unit Delay/1 -> Output/1, Sum/2, [SP17]
  Saturation/1 -> Unit Delay/1
  Vel PI/1(Delta Output) -> Sum/1
  Sum/1 -> Saturation/1

== system MultiLoop_mode3/TE Plant/Reactor pressure ==
  Setpoint : Inport
  Meas : Inport  Port=2
  Saturation : Saturate  UpperLimit=Hi  LowerLimit=Lo
  Sum : Sum  Inputs=|++  SaturateOnIntegerOverflow=on
  Unit Delay : UnitDelay  InitialCondition=x0  SampleTime=Ts
  Vel PI : Subsystem  mask{Kc=Kc, Ti=Ti, Ts=Ts}
  Output : Outport
  wires:
  Setpoint/1 -> Vel PI/1(Setpoint)
  Meas/1 -> Vel PI/2(Meas)
  Unit Delay/1 -> Output/1, Sum/2
  Saturation/1 -> Unit Delay/1
  Vel PI/1(Delta Output) -> Sum/1
  Sum/1 -> Saturation/1

== system MultiLoop_mode3/TE Plant/Recycle Valve Override ==
  Desired : Inport
  Coolant Valve % : Inport  Port=2
  Gain : Gain  Gain=-2
  Max Allowed : Constant  Value=90
  Saturation : Saturate  UpperLimit=100  LowerLimit=0
  Saturation1 : Saturate  UpperLimit=0  LowerLimit=-Inf
  Sum : Sum  Inputs=|+-  SaturateOnIntegerOverflow=on
  Sum1 : Sum  Inputs=++|
  Output : Outport  VectorParamsAs1DForOutWhenUnconnected=off
  wires:
  Saturation/1 -> Output/1
  Coolant Valve %/1 -> Sum/1
  Sum/1 -> Gain/1
  Max Allowed/1 -> Sum/2
  Gain/1 -> Saturation1/1
  Sum1/1 -> Saturation/1
  Saturation1/1 -> Sum1/2
  Desired/1 -> Sum1/1

== system MultiLoop_mode3/TE Plant/Separator flow rate ==
  Ratio : Inport
  Measured Flow : Inport  Port=2
  Discrete PI : TElib/Discrete PI  Kc=4e-4  Ti=0.001/60  Ts=Ts_base  x0=xmv_0(7)  Hi=100  Lo=0
      link override Vel PI/Goto: GotoTag=xmv7_integrator
      link override Vel PI/Unit Delay: InitialCondition=integrator_init(6)
  Product : Product  SaturateOnIntegerOverflow=on  OutDataTypeStr=Inherit: Same as first input
  Valve % : Outport  VectorParamsAs1DForOutWhenUnconnected=off
  wires:
  Product/1 -> Discrete PI/1
  Measured Flow/1 -> Discrete PI/2
  [Fp] -> Product/2
  Ratio/1 -> Product/1
  Discrete PI/1 -> Valve %/1

== system MultiLoop_mode3/TE Plant/Stripper flow rate ==
  Ratio : Inport
  Measured Flow : Inport  Port=2
  Discrete PI : TElib/Discrete PI  Kc=4e-4  Ti=0.001/60  Ts=Ts_base  x0=xmv_0(8)  Hi=100  Lo=0
      link override Vel PI/Goto: GotoTag=xmv8_integrator
      link override Vel PI/Unit Delay: InitialCondition=integrator_init(7)
  Product : Product  SaturateOnIntegerOverflow=on  OutDataTypeStr=Inherit: Same as first input
  Scope : Scope
  Valve % : Outport  VectorParamsAs1DForOutWhenUnconnected=off
  wires:
  Discrete PI/1 -> Scope/1, Valve %/1
  Ratio/1 -> Product/1
  [Fp] -> Product/2
  Measured Flow/1 -> Discrete PI/2
  Product/1 -> Discrete PI/1

== system MultiLoop_mode3/TE Plant/Stripper level ==
  Setpoint : Inport
  Meas : Inport  Port=2
  Saturation : Saturate  UpperLimit=Hi  LowerLimit=Lo
  Sum : Sum  Inputs=|++  SaturateOnIntegerOverflow=on
  Unit Delay : UnitDelay  InitialCondition=x0  SampleTime=Ts
  Vel PI : Subsystem  mask{Kc=Kc, Ti=Ti, Ts=Ts}
  Output : Outport
  wires:
  Setpoint/1 -> Vel PI/1(Setpoint)
  Meas/1 -> Vel PI/2(Meas)
  Unit Delay/1 -> Output/1, Sum/2
  Saturation/1 -> Unit Delay/1
  Vel PI/1(Delta Output) -> Sum/1
  Sum/1 -> Saturation/1

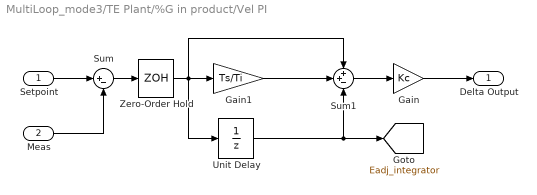
== system MultiLoop_mode3/TE Plant/%G in product/Vel PI ==
  Setpoint : Inport
  Meas : Inport  Port=2
  Gain : Gain  Gain=Kc  SaturateOnIntegerOverflow=on  OutDataTypeStr=Inherit: Same as input  ParamDataTypeStr=Inherit: Same as input
  Gain1 : Gain  Gain=Ts/Ti  SaturateOnIntegerOverflow=on  OutDataTypeStr=Inherit: Same as input  ParamDataTypeStr=Inherit: Same as input
  Sum : Sum  Inputs=|+-  SaturateOnIntegerOverflow=on
  Sum1 : Sum  Inputs=++-  SaturateOnIntegerOverflow=on
  Unit Delay : UnitDelay  InitialCondition=integrator_init(12)  SampleTime=Ts
  Zero-Order Hold : ZeroOrderHold  SampleTime=Ts
  Delta Output : Outport
  tag scope: Eadj_integrator=global
  wires:
  Zero-Order Hold/1 -> Sum1/1, Unit Delay/1, Gain1/1
  Sum/1 -> Zero-Order Hold/1
  Unit Delay/1 -> [Eadj_integrator], Sum1/3
  Gain1/1 -> Sum1/2
  Sum1/1 -> Gain/1
  Gain/1 -> Delta Output/1
  Meas/1 -> Sum/2
  Setpoint/1 -> Sum/1

== system MultiLoop_mode3/TE Plant/A feed rate/Discrete PI ==
  Setpoint : Inport
  Meas : Inport  Port=2
  Saturation : Saturate  UpperLimit=Hi  LowerLimit=Lo
  Sum : Sum  Inputs=|++  SaturateOnIntegerOverflow=on
  Unit Delay : UnitDelay  InitialCondition=x0  SampleTime=Ts
  Vel PI : Subsystem  mask{Kc=Kc, Ti=Ti, Ts=Ts}
  Output : Outport
  wires:
  Setpoint/1 -> Vel PI/1(Setpoint)
  Meas/1 -> Vel PI/2(Meas)
  Unit Delay/1 -> Output/1, Sum/2
  Saturation/1 -> Unit Delay/1
  Vel PI/1(Delta Output) -> Sum/1
  Sum/1 -> Saturation/1

== system MultiLoop_mode3/TE Plant/C feed rate/Discrete PI ==
  Setpoint : Inport
  Meas : Inport  Port=2
  Saturation : Saturate  UpperLimit=Hi  LowerLimit=Lo
  Scope : Scope
  Scope1 : Scope
  Sum : Sum  Inputs=|++  SaturateOnIntegerOverflow=on
  Unit Delay : UnitDelay  InitialCondition=x0  SampleTime=Ts
  Vel PI : Subsystem  mask{Kc=Kc, Ti=Ti, Ts=Ts}
  Output : Outport
  wires:
  Setpoint/1 -> Vel PI/1(Setpoint)
  Meas/1 -> Vel PI/2(Meas)
  Unit Delay/1 -> Output/1, Scope/1, Sum/2
  Saturation/1 -> Unit Delay/1
  Vel PI/1(Delta Output) -> Scope1/1, Sum/1
  Sum/1 -> Saturation/1

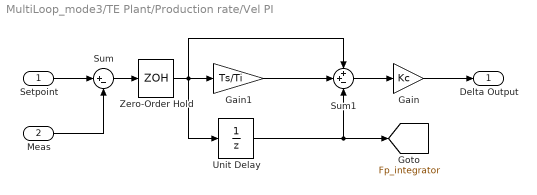
== system MultiLoop_mode3/TE Plant/Production rate/Vel PI ==
  Setpoint : Inport
  Meas : Inport  Port=2
  Gain : Gain  Gain=Kc  SaturateOnIntegerOverflow=on  OutDataTypeStr=Inherit: Same as input  ParamDataTypeStr=Inherit: Same as input
  Gain1 : Gain  Gain=Ts/Ti  SaturateOnIntegerOverflow=on  OutDataTypeStr=Inherit: Same as input  ParamDataTypeStr=Inherit: Same as input
  Sum : Sum  Inputs=|+-  SaturateOnIntegerOverflow=on
  Sum1 : Sum  Inputs=++-  SaturateOnIntegerOverflow=on
  Unit Delay : UnitDelay  InitialCondition=integrator_init(10)  SampleTime=Ts
  Zero-Order Hold : ZeroOrderHold  SampleTime=Ts
  Delta Output : Outport
  tag scope: Fp_integrator=global
  wires:
  Zero-Order Hold/1 -> Sum1/1, Unit Delay/1, Gain1/1
  Sum/1 -> Zero-Order Hold/1
  Unit Delay/1 -> [Fp_integrator], Sum1/3
  Gain1/1 -> Sum1/2
  Sum1/1 -> Gain/1
  Gain/1 -> Delta Output/1
  Meas/1 -> Sum/2
  Setpoint/1 -> Sum/1

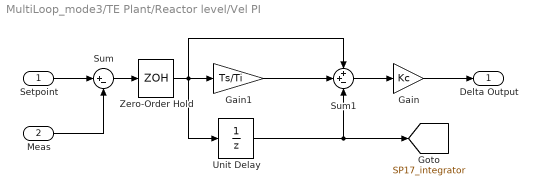
== system MultiLoop_mode3/TE Plant/Reactor level/Vel PI ==
  Setpoint : Inport
  Meas : Inport  Port=2
  Gain : Gain  Gain=Kc  SaturateOnIntegerOverflow=on  OutDataTypeStr=Inherit: Same as input  ParamDataTypeStr=Inherit: Same as input
  Gain1 : Gain  Gain=Ts/Ti  SaturateOnIntegerOverflow=on  OutDataTypeStr=Inherit: Same as input  ParamDataTypeStr=Inherit: Same as input
  Sum : Sum  Inputs=|+-  SaturateOnIntegerOverflow=on
  Sum1 : Sum  Inputs=++-  SaturateOnIntegerOverflow=on
  Unit Delay : UnitDelay  InitialCondition=integrator_init(11)  SampleTime=Ts
  Zero-Order Hold : ZeroOrderHold  SampleTime=Ts
  Delta Output : Outport
  tag scope: SP17_integrator=global
  wires:
  Zero-Order Hold/1 -> Sum1/1, Unit Delay/1, Gain1/1
  Sum/1 -> Zero-Order Hold/1
  Unit Delay/1 -> Sum1/3, [SP17_integrator]
  Gain1/1 -> Sum1/2
  Sum1/1 -> Gain/1
  Gain/1 -> Delta Output/1
  Meas/1 -> Sum/2
  Setpoint/1 -> Sum/1

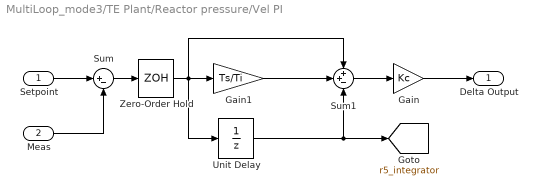
== system MultiLoop_mode3/TE Plant/Reactor pressure/Vel PI ==
  Setpoint : Inport
  Meas : Inport  Port=2
  Gain : Gain  Gain=Kc  SaturateOnIntegerOverflow=on  OutDataTypeStr=Inherit: Same as input  ParamDataTypeStr=Inherit: Same as input
  Gain1 : Gain  Gain=Ts/Ti  SaturateOnIntegerOverflow=on  OutDataTypeStr=Inherit: Same as input  ParamDataTypeStr=Inherit: Same as input
  Sum : Sum  Inputs=|+-  SaturateOnIntegerOverflow=on
  Sum1 : Sum  Inputs=++-  SaturateOnIntegerOverflow=on
  Unit Delay : UnitDelay  InitialCondition=integrator_init(13)  SampleTime=Ts
  Zero-Order Hold : ZeroOrderHold  SampleTime=Ts
  Delta Output : Outport
  tag scope: r5_integrator=global
  wires:
  Zero-Order Hold/1 -> Sum1/1, Unit Delay/1, Gain1/1
  Sum/1 -> Zero-Order Hold/1
  Unit Delay/1 -> [r5_integrator], Sum1/3
  Gain1/1 -> Sum1/2
  Sum1/1 -> Gain/1
  Gain/1 -> Delta Output/1
  Meas/1 -> Sum/2
  Setpoint/1 -> Sum/1

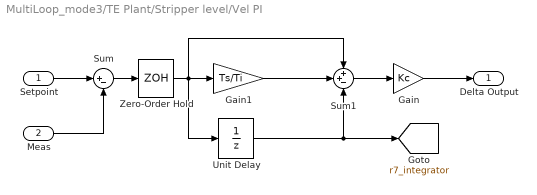
== system MultiLoop_mode3/TE Plant/Stripper level/Vel PI ==
  Setpoint : Inport
  Meas : Inport  Port=2
  Gain : Gain  Gain=Kc  SaturateOnIntegerOverflow=on  OutDataTypeStr=Inherit: Same as input  ParamDataTypeStr=Inherit: Same as input
  Gain1 : Gain  Gain=Ts/Ti  SaturateOnIntegerOverflow=on  OutDataTypeStr=Inherit: Same as input  ParamDataTypeStr=Inherit: Same as input
  Sum : Sum  Inputs=|+-  SaturateOnIntegerOverflow=on
  Sum1 : Sum  Inputs=++-  SaturateOnIntegerOverflow=on
  Unit Delay : UnitDelay  InitialCondition=integrator_init(15)  SampleTime=Ts
  Zero-Order Hold : ZeroOrderHold  SampleTime=Ts
  Delta Output : Outport
  tag scope: r7_integrator=global
  wires:
  Zero-Order Hold/1 -> Sum1/1, Unit Delay/1, Gain1/1
  Sum/1 -> Zero-Order Hold/1
  Unit Delay/1 -> [r7_integrator], Sum1/3
  Gain1/1 -> Sum1/2
  Sum1/1 -> Gain/1
  Gain/1 -> Delta Output/1
  Meas/1 -> Sum/2
  Setpoint/1 -> Sum/1

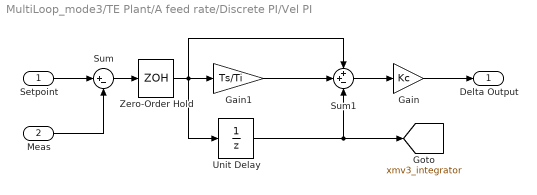
== system MultiLoop_mode3/TE Plant/A feed rate/Discrete PI/Vel PI ==
  Setpoint : Inport
  Meas : Inport  Port=2
  Gain : Gain  Gain=Kc  SaturateOnIntegerOverflow=on  OutDataTypeStr=Inherit: Same as input  ParamDataTypeStr=Inherit: Same as input
  Gain1 : Gain  Gain=Ts/Ti  SaturateOnIntegerOverflow=on  OutDataTypeStr=Inherit: Same as input  ParamDataTypeStr=Inherit: Same as input
  Sum : Sum  Inputs=|+-  SaturateOnIntegerOverflow=on
  Sum1 : Sum  Inputs=++-  SaturateOnIntegerOverflow=on
  Unit Delay : UnitDelay  InitialCondition=integrator_init(3)  SampleTime=Ts
  Zero-Order Hold : ZeroOrderHold  SampleTime=Ts
  Delta Output : Outport
  tag scope: xmv3_integrator=global
  wires:
  Zero-Order Hold/1 -> Sum1/1, Unit Delay/1, Gain1/1
  Sum/1 -> Zero-Order Hold/1
  Unit Delay/1 -> Sum1/3, [xmv3_integrator]
  Gain1/1 -> Sum1/2
  Sum1/1 -> Gain/1
  Gain/1 -> Delta Output/1
  Meas/1 -> Sum/2
  Setpoint/1 -> Sum/1

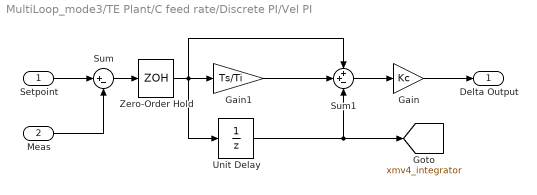
== system MultiLoop_mode3/TE Plant/C feed rate/Discrete PI/Vel PI ==
  Setpoint : Inport
  Meas : Inport  Port=2
  Gain : Gain  Gain=Kc  SaturateOnIntegerOverflow=on  OutDataTypeStr=Inherit: Same as input  ParamDataTypeStr=Inherit: Same as input
  Gain1 : Gain  Gain=Ts/Ti  SaturateOnIntegerOverflow=on  OutDataTypeStr=Inherit: Same as input  ParamDataTypeStr=Inherit: Same as input
  Sum : Sum  Inputs=|+-  SaturateOnIntegerOverflow=on
  Sum1 : Sum  Inputs=++-  SaturateOnIntegerOverflow=on
  Unit Delay : UnitDelay  InitialCondition=100  SampleTime=Ts
  Zero-Order Hold : ZeroOrderHold  SampleTime=Ts
  Delta Output : Outport
  tag scope: xmv4_integrator=global
  wires:
  Zero-Order Hold/1 -> Sum1/1, Unit Delay/1, Gain1/1
  Sum/1 -> Zero-Order Hold/1
  Unit Delay/1 -> Sum1/3, [xmv4_integrator]
  Gain1/1 -> Sum1/2
  Sum1/1 -> Gain/1
  Gain/1 -> Delta Output/1
  Meas/1 -> Sum/2
  Setpoint/1 -> Sum/1
